simulink model "MUTUAL_INDUCTANCE_SIMULINK"  (R2022b)
settings: Solver=ode4  StartTime=0.0  StopTime=10.0  FixedStep=StepSize  RelTol=1e-3
values from neighbouring files (symbols this model uses):
  L1 = 2    [MUTUAL_INDUCTANCE_SCRIPT.m]
  L2 = 2    [MUTUAL_INDUCTANCE_SCRIPT.m]
  M = 0.8    [MUTUAL_INDUCTANCE_SCRIPT.m]
  PhaseAngle = deg2rad(90)    [MUTUAL_INDUCTANCE_SCRIPT.m]
  R1 = 1    [MUTUAL_INDUCTANCE_SCRIPT.m]
  R2 = 0.5    [MUTUAL_INDUCTANCE_SCRIPT.m]
  Um = sqrt(2)*U    [MUTUAL_INDUCTANCE_SCRIPT.m]
  w = 2*pi*f    (= 314.159265359)    [MUTUAL_INDUCTANCE_SCRIPT.m]
settings Model: Creator=irfan  LastModifiedBy=irfan

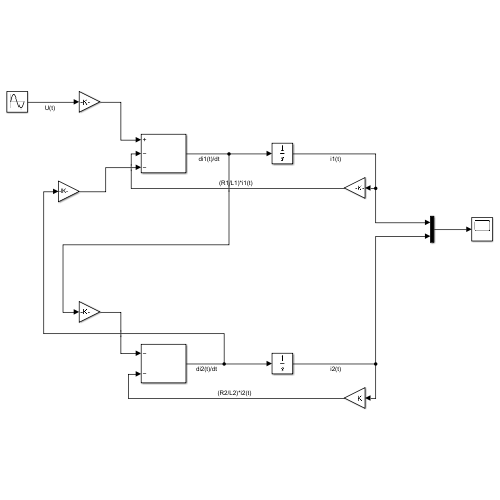
[thumbnail: Simulink's stored preview of the top-level diagram]
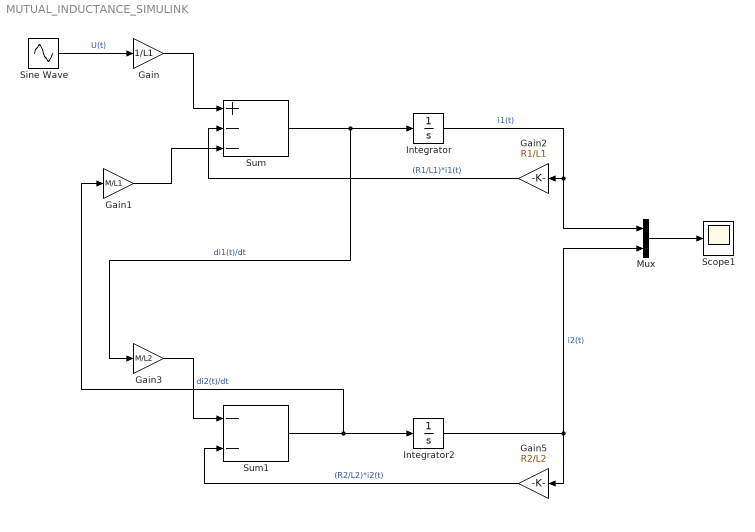
== system MUTUAL_INDUCTANCE_SIMULINK ==
  Gain : Gain  Gain=1/L1
  Gain1 : Gain  Gain=M/L1
  Gain2 : Gain  Gain=R1/L1
  Gain3 : Gain  Gain=M/L2
  Gain5 : Gain  Gain=R2/L2
  Integrator : Integrator
  Integrator2 : Integrator
  Mux : Mux  Inputs=2
  Scope1 : Scope
  Sine Wave : Sin  Amplitude=Um  Frequency=w  Phase=PhaseAngle  SampleTime=0
  Sum : Sum  Inputs=+--
  Sum1 : Sum  Inputs=--
  wires:
  Gain/1 -> Sum/1
  Sine Wave/1 -> Gain/1  "U(t)"
  Sum/1 -> Gain3/1, Integrator/1  "di1(t)/dt"
  Integrator/1 -> Mux/1, Gain2/1  "i1(t)"
  Gain2/1 -> Sum/2  "(R1/L1)*i1(t)"
  Sum1/1 -> Gain1/1, Integrator2/1  "di2(t)/dt"
  Integrator2/1 -> Mux/2, Gain5/1  "i2(t)"
  Gain5/1 -> Sum1/2  "(R2/L2)*i2(t)"
  Gain3/1 -> Sum1/1
  Gain1/1 -> Sum/3
  Mux/1 -> Scope1/1
